simulink model "gm_multi_module_phase_shift_generator_built_in_pwm"  (R2025b)
settings: Solver=FixedStepDiscrete  StartTime=0.0  StopTime=10e3  RelTol=1e-3
libraries: simulink x6, hdlsllib x3
settings Model: Creator=KoayXianCong  LastModifiedBy=KoayXianCong
settings OptimizationCC: BlockReduction=off  ConditionallyExecuteInputs=off  DefaultParameterBehavior=Inlined  InheritOutputTypeSmallerThanSingle=on
settings DebuggingCC: SignalRangeChecking=warning  ArtificialAlgebraicLoopMsg=error  InheritedTsInSrcMsg=none  SingleTaskRateTransMsg=error
settings HardwareCC: ProdBitPerPointer=32.0  ProdBitPerSizeT=32.0  ProdBitPerPtrDiffT=32.0  ProdLargestAtomicFloat=None  ProdIntDivRoundTo=Undefined  ProdEndianess=Unspecified  ProdWordSize=32.0  ProdHWDeviceType=ASIC/FPGA->ASIC/FPGA  TargetBitPerPointer=64.0  TargetBitPerSizeT=64.0  TargetBitPerPtrDiffT=64.0  TargetLongLongMode=on  TargetIntDivRoundTo=Zero  TargetEndianess=LittleEndian  TargetWordSize=64.0  TargetHWDeviceType=Custom Processor->MATLAB Host Computer  ProdEqTarget=off

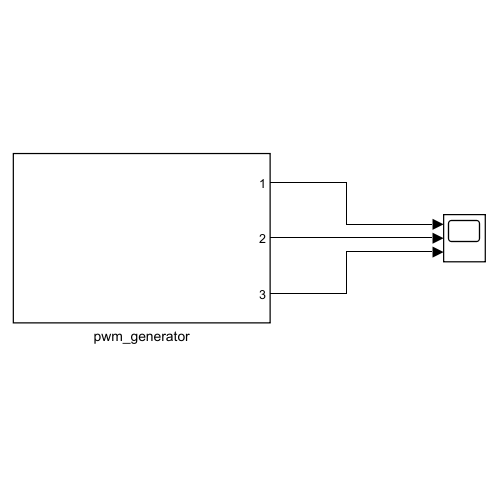
[thumbnail: Simulink's stored preview of the top-level diagram]
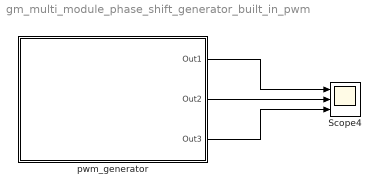
== system gm_multi_module_phase_shift_generator_built_in_pwm ==
  Scope4 : Scope  NumInputPorts=3
      settings: ActiveDisplayYMinimum=-0.12499999999999997  ActiveDisplayYMaximum=1.125  DataLoggingVariableName=ScopeData4  DataLoggingSaveFormat=Array
  pwm_generator : Subsystem
  wires:
  pwm_generator/3(Out3) -> Scope4/3
  pwm_generator/2(Out2) -> Scope4/2
  pwm_generator/1(Out1) -> Scope4/1

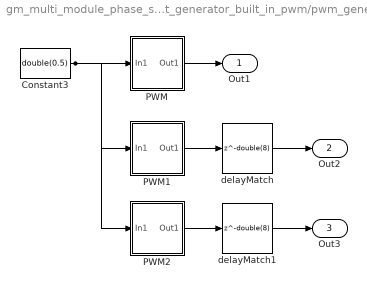
== system gm_multi_module_phase_shift_generator_built_in_pwm/pwm_generator ==
  Constant3 : Constant  Value=double(0.5)  VectorParams1D=off  OutDataTypeStr=double  SampleTime=1
  PWM : Subsystem
  PWM1 : Subsystem
  PWM2 : Subsystem
  delayMatch : Delay  DelayLength=double(8)  InitialCondition=0  SampleTime=1
  delayMatch1 : Delay  DelayLength=double(8)  InitialCondition=0  SampleTime=1
  Out1 : Outport  SampleTime=1
  Out2 : Outport  Port=2  SampleTime=1
  Out3 : Outport  Port=3  SampleTime=1
  wires:
  Constant3/1 -> PWM2/1(In1), PWM1/1(In1), PWM/1(In1)
  PWM/1(Out1) -> Out1/1
  PWM1/1(Out1) -> delayMatch/1
  PWM2/1(Out1) -> delayMatch1/1
  delayMatch1/1 -> Out3/1
  delayMatch/1 -> Out2/1

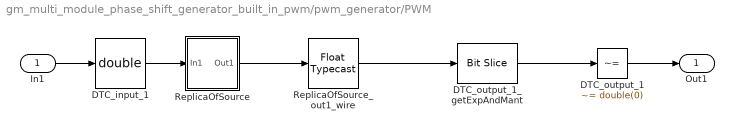
== system gm_multi_module_phase_shift_generator_built_in_pwm/pwm_generator/PWM ==
  In1 : Inport  OutDataTypeStr=double  PortDimensions=1  SampleTime=1  LockScale=on
  DTC_input_1 : DataTypeConversion  OutDataTypeStr=double
  DTC_output_1 : simulink/Logic and Bit Operations/Compare To Constant  relop=~=  const=double(0)  OutDataTypeStr=boolean
  DTC_output_1_getExpAndMant : hdlsllib/Logic and Bit Operations/Bit Slice  lidx=double(62)  ridx=double(0)
  ReplicaOfSource : Subsystem
  ReplicaOfSource_out1_wire : FloatTypecast
  Out1 : Outport  SampleTime=1  LockScale=on
  wires:
  DTC_output_1/1 -> Out1/1
  In1/1 -> DTC_input_1/1
  ReplicaOfSource/1(Out1) -> ReplicaOfSource_out1_wire/1
  DTC_input_1/1 -> ReplicaOfSource/1(In1)
  ReplicaOfSource_out1_wire/1 -> DTC_output_1_getExpAndMant/1
  DTC_output_1_getExpAndMant/1 -> DTC_output_1/1

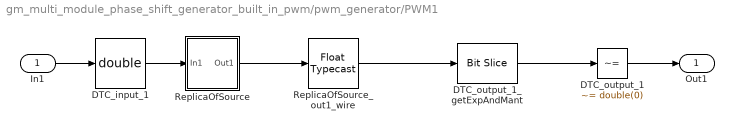
== system gm_multi_module_phase_shift_generator_built_in_pwm/pwm_generator/PWM1 ==
  In1 : Inport  OutDataTypeStr=double  PortDimensions=1  SampleTime=1  LockScale=on
  DTC_input_1 : DataTypeConversion  OutDataTypeStr=double
  DTC_output_1 : simulink/Logic and Bit Operations/Compare To Constant  relop=~=  const=double(0)  OutDataTypeStr=boolean
  DTC_output_1_getExpAndMant : hdlsllib/Logic and Bit Operations/Bit Slice  lidx=double(62)  ridx=double(0)
  ReplicaOfSource : Subsystem
  ReplicaOfSource_out1_wire : FloatTypecast
  Out1 : Outport  SampleTime=1  LockScale=on
  wires:
  DTC_output_1/1 -> Out1/1
  In1/1 -> DTC_input_1/1
  DTC_output_1_getExpAndMant/1 -> DTC_output_1/1
  DTC_input_1/1 -> ReplicaOfSource/1(In1)
  ReplicaOfSource/1(Out1) -> ReplicaOfSource_out1_wire/1
  ReplicaOfSource_out1_wire/1 -> DTC_output_1_getExpAndMant/1

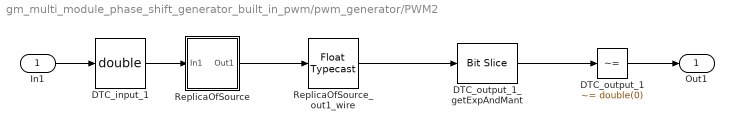
== system gm_multi_module_phase_shift_generator_built_in_pwm/pwm_generator/PWM2 ==
  In1 : Inport  OutDataTypeStr=double  PortDimensions=1  SampleTime=1  LockScale=on
  DTC_input_1 : DataTypeConversion  OutDataTypeStr=double
  DTC_output_1 : simulink/Logic and Bit Operations/Compare To Constant  relop=~=  const=double(0)  OutDataTypeStr=boolean
  DTC_output_1_getExpAndMant : hdlsllib/Logic and Bit Operations/Bit Slice  lidx=double(62)  ridx=double(0)
  ReplicaOfSource : Subsystem
  ReplicaOfSource_out1_wire : FloatTypecast
  Out1 : Outport  SampleTime=1  LockScale=on
  wires:
  In1/1 -> DTC_input_1/1
  DTC_output_1/1 -> Out1/1
  DTC_input_1/1 -> ReplicaOfSource/1(In1)
  ReplicaOfSource/1(Out1) -> ReplicaOfSource_out1_wire/1
  ReplicaOfSource_out1_wire/1 -> DTC_output_1_getExpAndMant/1
  DTC_output_1_getExpAndMant/1 -> DTC_output_1/1

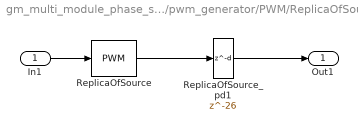
== system gm_multi_module_phase_shift_generator_built_in_pwm/pwm_generator/PWM/ReplicaOfSource ==
  In1 : Inport
  ReplicaOfSource : simulink/Discontinuities/PWM  DisableCoverage=on  Period=1024  InitialDelay=0  DisallowZeroDutyCycle=on  RunAtFixedTimeIntervals=on  SampleTime=1
      settings: LibrarySourceBlock=hdlsllib/RCP and HIL/PWM
  ReplicaOfSource_pd1 : Delay  DelayLength=26
  Out1 : Outport
  wires:
  ReplicaOfSource/1 -> ReplicaOfSource_pd1/1
  In1/1 -> ReplicaOfSource/1
  ReplicaOfSource_pd1/1 -> Out1/1

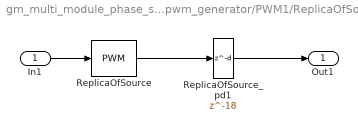
== system gm_multi_module_phase_shift_generator_built_in_pwm/pwm_generator/PWM1/ReplicaOfSource ==
  In1 : Inport
  ReplicaOfSource : simulink/Discontinuities/PWM  DisableCoverage=on  Period=1024  InitialDelay=1024/3  DisallowZeroDutyCycle=on  RunAtFixedTimeIntervals=on  SampleTime=1
      settings: LibrarySourceBlock=hdlsllib/RCP and HIL/PWM
  ReplicaOfSource_pd1 : Delay  DelayLength=18
  Out1 : Outport
  wires:
  ReplicaOfSource_pd1/1 -> Out1/1
  In1/1 -> ReplicaOfSource/1
  ReplicaOfSource/1 -> ReplicaOfSource_pd1/1

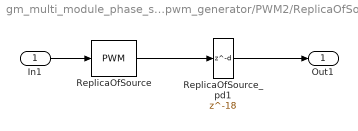
== system gm_multi_module_phase_shift_generator_built_in_pwm/pwm_generator/PWM2/ReplicaOfSource ==
  In1 : Inport
  ReplicaOfSource : simulink/Discontinuities/PWM  DisableCoverage=on  Period=1024  InitialDelay=(2*1024)/3  DisallowZeroDutyCycle=off  RunAtFixedTimeIntervals=on  SampleTime=1
      settings: LibrarySourceBlock=hdlsllib/RCP and HIL/PWM
  ReplicaOfSource_pd1 : Delay  DelayLength=18
  Out1 : Outport
  wires:
  In1/1 -> ReplicaOfSource/1
  ReplicaOfSource/1 -> ReplicaOfSource_pd1/1
  ReplicaOfSource_pd1/1 -> Out1/1
